simulink model "embc_proj"  (R2025b)
settings: Solver=VariableStepAuto  StartTime=0.0  StopTime=10.0  RelTol=1e-3
libraries: simulink x2, dspinverses x1
settings Model: Creator=lenovo  LastModifiedBy=lenovo
settings DebuggingCC: AlgebraicLoopMsg=none

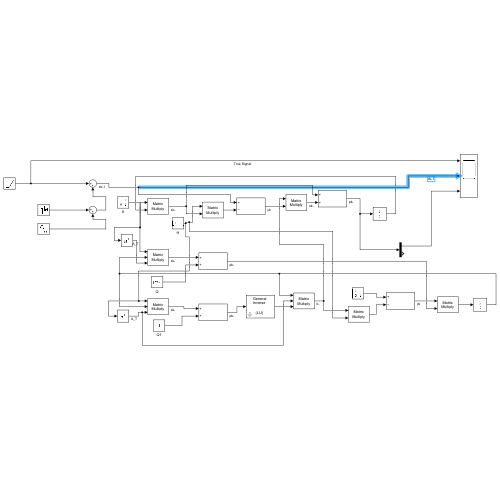
[thumbnail: Simulink's stored preview of the top-level diagram]
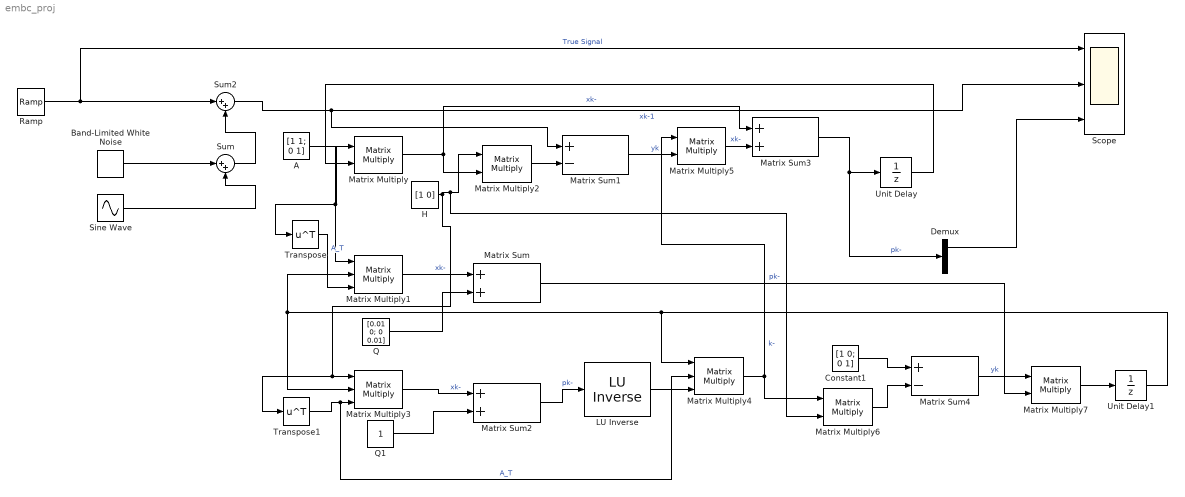
== system embc_proj ==
  " LU Inverse" : dspinverses/ LU Inverse
  A : Constant  Value=[1 1; 0 1]  VectorParams1D=off
  Band-Limited White Noise : simulink/Sources/Band-Limited White Noise  Cov=[0.1]  Ts=0.1  seed=[23341]
  Constant1 : Constant  Value=[1 0; 0 1]  VectorParams1D=off
  Demux : Demux  Outputs=2
  H : Constant  Value=[1 0]  VectorParams1D=off
  Matrix Sum : Sum
  Matrix Sum1 : Sum  Inputs=+-
  Matrix Sum2 : Sum
  Matrix Sum3 : Sum
  Matrix Sum4 : Sum  Inputs=+-
  Matrix Multiply{,2,5..7} (5 alike) : Product  Multiplication=Matrix(*)
  Matrix Multiply1 : Product  Inputs=3  Multiplication=Matrix(*)
  Matrix Multiply3 : Product  Inputs=3  Multiplication=Matrix(*)
  Matrix Multiply4 : Product  Inputs=3  Multiplication=Matrix(*)
  Q : Constant  Value=[0.01 0; 0 0.01]  VectorParams1D=off
  Q1 : Constant  VectorParams1D=off
  Ramp : simulink/Sources/Ramp  slope=4  start=0  InitialOutput=0
  Scope : Scope  NumInputPorts=3
      settings: ActiveDisplayYMinimum=-5.2055654282630668  ActiveDisplayYMaximum=46.850088854367613
  Sine Wave : Sin  Amplitude=0.98  SampleTime=0
  Sum : Sum  Inputs=|++
  Sum2 : Sum  Inputs=|++
  Transpose : Math  Operator=transpose
  Transpose1 : Math  Operator=transpose
  Unit Delay : UnitDelay  SampleTime=-1  HasFrameUpgradeWarning=on
  Unit Delay1 : UnitDelay  SampleTime=-1  HasFrameUpgradeWarning=on
  wires:
  Ramp/1 -> Scope/1, Sum2/1  "True Signal"
  Band-Limited White Noise/1 -> Sum/1
  Sum/1 -> Sum2/2
  Sum2/1 -> Matrix Sum1/1, Scope/2  "xk-1"
  Sine Wave/1 -> Sum/2
  A/1 -> Transpose/1, Matrix Multiply/1, Matrix Multiply1/1
  Transpose/1 -> Matrix Multiply1/3  "A_T"
  Matrix Multiply1/1 -> Matrix Sum/1  "xk-"
  Q/1 -> Matrix Sum/2
  Matrix Multiply2/1 -> Matrix Sum1/2
  Transpose1/1 -> Matrix Multiply4/2, Matrix Multiply3/3  "A_T"
  Matrix Multiply3/1 -> Matrix Sum2/1  "xk-"
  Q1/1 -> Matrix Sum2/2
  Matrix Sum2/1 -> " LU Inverse"/1  "pk-"
  " LU Inverse"/1 -> Matrix Multiply4/3
  Matrix Multiply4/1 -> Matrix Multiply6/1, Matrix Multiply5/1  "k-"
  Matrix Sum1/1 -> Matrix Multiply5/2  "yk"
  Matrix Multiply5/1 -> Matrix Sum3/2  "xk-"
  Unit Delay1/1 -> Matrix Multiply1/2, Matrix Multiply3/2, Matrix Multiply4/1
  Matrix Multiply/1 -> Matrix Multiply2/2, Matrix Sum3/1  "xk-"
  Matrix Sum3/1 -> Demux/1, Unit Delay/1  "pk-"
  Unit Delay/1 -> Matrix Multiply/2
  Demux/1 -> Scope/3
  Constant1/1 -> Matrix Sum4/1
  Matrix Multiply6/1 -> Matrix Sum4/2
  H/1 -> Matrix Multiply6/2, Matrix Multiply2/1, Transpose1/1, Matrix Multiply3/1
  Matrix Sum4/1 -> Matrix Multiply7/1  "yk"
  Matrix Sum/1 -> Matrix Multiply7/2  "pk-"
  Matrix Multiply7/1 -> Unit Delay1/1
